simulink model "Final_System_Model_V10"  (R2018a)
settings: Solver=VariableStepAuto  StartTime=0  StopTime=250  FixedStep=0.5  RelTol=1e-3
PreLoadFcn:
  | Ts_Power=1e-6;
  | Ts_Control=100e-6;
undefined symbols (not defined in the file): DiscIntNeverNeededParam, sigbuilder_block
libraries: simulink x24, fl_lib x16, powerlib x15, nesl_utility x8, powerlib_meascontrol x5, re_lib x1
(part 8 of 8)

== system Final_System_Model_V10/Full System/Electrolysers/260 KW Electrolyzer Stack_1/electrolyser stack/electrolyser cell/Eta_B/segma_B/Beta ==
  In1 : Inport
  In2 : Inport  Port=2
  Add3 : Sum
  Add4 : Sum  Inputs=-+
  Add5 : Sum  Inputs=+-
  Add6 : Sum  Inputs=-+
  Constant3 : Constant
  Constant4 : Constant  Value=4
  Constant5 : Constant  Value=2
  Math Function1 : Math  Operator=square  SaturateOnIntegerOverflow=on
  Product5 : Product  Inputs=***
  Product6 : Product  Inputs=*/
  Product7 : Product  Inputs=*/
  Product8 : Product  Inputs=**
  Sqrt : Sqrt  SaturateOnIntegerOverflow=on
  Out1 : Outport
  wires:
  Math Function1/1 -> Add4/2
  Constant3/1 -> Product6/1, Add5/1, Add3/1
  Add3/1 -> Add6/2, Math Function1/1
  Sqrt/1 -> Add6/1
  Constant4/1 -> Product5/1
  Constant5/1 -> Product8/2
  Add4/1 -> Sqrt/1
  Product6/1 -> Add5/2
  Product5/1 -> Add4/1
  Add6/1 -> Product7/1
  Product8/1 -> Product7/2
  Product7/1 -> Out1/1
  In1/1 -> Product5/2, Add3/2
  In2/1 -> Product6/2
  Add5/1 -> Product8/1, Product5/3

== system Final_System_Model_V10/Full System/Electrolysers/260 KW Electrolyzer Stack_1/electrolyser stack/electrolyser cell/Eta_B/segma_B/K_a ==
  In1 : Inport
  In2 : Inport  Port=2
  In3 : Inport  Port=3
  Add2 : Sum  Inputs=+-
  Constant : Constant  Value=-523000
  Constant1 : Constant
  Math Function : Math  SaturateOnIntegerOverflow=on
  Product2 : Product  Inputs=*/
  Product3 : Product  Inputs=*/
  Product4 : Product
  Out1 : Outport
  Out2 : Outport  Port=2
  wires:
  Product4/1 -> Math Function/1
  Add2/1 -> Out2/1, Product4/2
  Math Function/1 -> Out1/1
  In3/1 -> Add2/2
  In2/1 -> Product3/2
  Product2/1 -> Product4/1
  Constant1/1 -> Product3/1
  Product3/1 -> Add2/1
  Constant/1 -> Product2/1
  In1/1 -> Product2/2

== system Final_System_Model_V10/Full System/Electrolysers/260 KW Electrolyzer Stack_1/electrolyser stack/electrolyser cell/Eta_B/segma_B/eta_B ==
  In1 : Inport
  In2 : Inport  Port=2
  Add : Sum
  Product : Product  Inputs=*/
  Out1 : Outport
  wires:
  Product/1 -> Out1/1
  In2/1 -> Add/2
  In1/1 -> Product/1, Add/1
  Add/1 -> Product/2

== system Final_System_Model_V10/Full System/Electrolysers/260 KW Electrolyzer Stack_1/electrolyser stack/electrolyser cell/Eta_B/segma_B/eta_B0 ==
  In1 : Inport
  In2 : Inport  Port=2
  Add1 : Sum
  Product1 : Product  Inputs=/*
  Out1 : Outport
  wires:
  Add1/1 -> Product1/1
  Product1/1 -> Out1/1
  In1/1 -> Add1/1
  In2/1 -> Product1/2, Add1/2

== system Final_System_Model_V10/Full System/Electrolysers/260 KW Electrolyzer Stack_1/electrolyser stack/electrolyser cell/eta_a/n_a/i_a0 ==
  In1 : Inport
  In2 : Inport  Port=2
  Divide : Product  Inputs=*/
  E_a : Constant  Value=76
  Exp : Math  SaturateOnIntegerOverflow=on
  Gain : Gain  Gain=-1
  Multiply : Product
  Multiply1 : Product  Inputs=3
  i_a0ref : Constant  Value=5e-12
  lamda_ma : Subsystem
  Out1 : Outport
  wires:
  Gain/1 -> Exp/1
  Exp/1 -> Multiply1/3
  Multiply/1 -> Gain/1
  Divide/1 -> Multiply/1
  i_a0ref/1 -> Multiply1/1
  In2/1 -> Multiply/2
  Multiply1/1 -> Out1/1
  E_a/1 -> Divide/1
  lamda_ma/1(Out1) -> Multiply1/2
  In1/1 -> Divide/2

== system Final_System_Model_V10/Full System/Electrolysers/260 KW Electrolyzer Stack_1/electrolyser stack/electrolyser cell/eta_c/n_c/i_c0 ==
  In1 : Inport
  In2 : Inport  Port=2
  Divide : Product  Inputs=*/
  E_c : Constant  Value=4.3
  Exp : Math  SaturateOnIntegerOverflow=on
  Gain : Gain  Gain=-1
  Multiply : Product  Inputs=3
  Multiply1 : Product
  i_c0ref : Constant  Value=1e-3
  lamda_mc : Subsystem
  Out1 : Outport
  wires:
  i_c0ref/1 -> Multiply/2
  Multiply/1 -> Out1/1
  Divide/1 -> Multiply1/2
  Multiply1/1 -> Gain/1
  E_c/1 -> Divide/1
  In1/1 -> Divide/2
  lamda_mc/1(Out1) -> Multiply/1
  Exp/1 -> Multiply/3
  Gain/1 -> Exp/1
  In2/1 -> Multiply1/1

== system Final_System_Model_V10/Full System/Electrolysers/93 KW Electrolyzer Stack_2/electrolyser stack/electrolyser cell/Eta_B/segma_B/Beta ==
  In1 : Inport
  In2 : Inport  Port=2
  Add3 : Sum
  Add4 : Sum  Inputs=-+
  Add5 : Sum  Inputs=+-
  Add6 : Sum  Inputs=-+
  Constant3 : Constant
  Constant4 : Constant  Value=4
  Constant5 : Constant  Value=2
  Math Function1 : Math  Operator=square  SaturateOnIntegerOverflow=on
  Product5 : Product  Inputs=***
  Product6 : Product  Inputs=*/
  Product7 : Product  Inputs=*/
  Product8 : Product  Inputs=**
  Sqrt : Sqrt  SaturateOnIntegerOverflow=on
  Out1 : Outport
  wires:
  Add5/1 -> Product5/3, Product8/1
  In2/1 -> Product6/2
  In1/1 -> Add3/2, Product5/2
  Product7/1 -> Out1/1
  Product8/1 -> Product7/2
  Add6/1 -> Product7/1
  Product5/1 -> Add4/1
  Product6/1 -> Add5/2
  Add4/1 -> Sqrt/1
  Constant5/1 -> Product8/2
  Constant4/1 -> Product5/1
  Sqrt/1 -> Add6/1
  Add3/1 -> Math Function1/1, Add6/2
  Constant3/1 -> Add3/1, Add5/1, Product6/1
  Math Function1/1 -> Add4/2

== system Final_System_Model_V10/Full System/Electrolysers/93 KW Electrolyzer Stack_2/electrolyser stack/electrolyser cell/Eta_B/segma_B/K_a ==
  In1 : Inport
  In2 : Inport  Port=2
  In3 : Inport  Port=3
  Add2 : Sum  Inputs=+-
  Constant : Constant  Value=-523000
  Constant1 : Constant
  Math Function : Math  SaturateOnIntegerOverflow=on
  Product2 : Product  Inputs=*/
  Product3 : Product  Inputs=*/
  Product4 : Product
  Out1 : Outport
  Out2 : Outport  Port=2
  wires:
  In1/1 -> Product2/2
  Constant/1 -> Product2/1
  Product3/1 -> Add2/1
  Constant1/1 -> Product3/1
  Product2/1 -> Product4/1
  In2/1 -> Product3/2
  In3/1 -> Add2/2
  Math Function/1 -> Out1/1
  Add2/1 -> Product4/2, Out2/1
  Product4/1 -> Math Function/1

== system Final_System_Model_V10/Full System/Electrolysers/93 KW Electrolyzer Stack_2/electrolyser stack/electrolyser cell/Eta_B/segma_B/eta_B ==
  In1 : Inport
  In2 : Inport  Port=2
  Add : Sum
  Product : Product  Inputs=*/
  Out1 : Outport
  wires:
  Add/1 -> Product/2
  In1/1 -> Add/1, Product/1
  In2/1 -> Add/2
  Product/1 -> Out1/1

== system Final_System_Model_V10/Full System/Electrolysers/93 KW Electrolyzer Stack_2/electrolyser stack/electrolyser cell/Eta_B/segma_B/eta_B0 ==
  In1 : Inport
  In2 : Inport  Port=2
  Add1 : Sum
  Product1 : Product  Inputs=/*
  Out1 : Outport
  wires:
  In2/1 -> Add1/2, Product1/2
  In1/1 -> Add1/1
  Product1/1 -> Out1/1
  Add1/1 -> Product1/1

== system Final_System_Model_V10/Full System/Electrolysers/93 KW Electrolyzer Stack_2/electrolyser stack/electrolyser cell/eta_a/n_a/i_a0 ==
  In1 : Inport
  In2 : Inport  Port=2
  Divide : Product  Inputs=*/
  E_a : Constant  Value=76
  Exp : Math  SaturateOnIntegerOverflow=on
  Gain : Gain  Gain=-1
  Multiply : Product
  Multiply1 : Product  Inputs=3
  i_a0ref : Constant  Value=5e-12
  lamda_ma : Subsystem
  Out1 : Outport
  wires:
  In1/1 -> Divide/2
  lamda_ma/1(Out1) -> Multiply1/2
  E_a/1 -> Divide/1
  Multiply1/1 -> Out1/1
  In2/1 -> Multiply/2
  i_a0ref/1 -> Multiply1/1
  Divide/1 -> Multiply/1
  Multiply/1 -> Gain/1
  Exp/1 -> Multiply1/3
  Gain/1 -> Exp/1

== system Final_System_Model_V10/Full System/Electrolysers/93 KW Electrolyzer Stack_2/electrolyser stack/electrolyser cell/eta_c/n_c/i_c0 ==
  In1 : Inport
  In2 : Inport  Port=2
  Divide : Product  Inputs=*/
  E_c : Constant  Value=4.3
  Exp : Math  SaturateOnIntegerOverflow=on
  Gain : Gain  Gain=-1
  Multiply : Product  Inputs=3
  Multiply1 : Product
  i_c0ref : Constant  Value=1e-3
  lamda_mc : Subsystem
  Out1 : Outport
  wires:
  In2/1 -> Multiply1/1
  Gain/1 -> Exp/1
  Exp/1 -> Multiply/3
  lamda_mc/1(Out1) -> Multiply/1
  In1/1 -> Divide/2
  E_c/1 -> Divide/1
  Multiply1/1 -> Gain/1
  Divide/1 -> Multiply1/2
  Multiply/1 -> Out1/1
  i_c0ref/1 -> Multiply/2

== system Final_System_Model_V10/Full System/Subsystem1/100KW Fuel Cell Stack_2/Fuel Cell Model/ From Current Density (A//cm^2) To Overvoltages (V)/Concentration Overvoltage/IF Function/If Action Subsystem ==
  In1 : Inport
  Action Port : ActionPort  ActionType=then
  Math Function1 : Math  Operator=log  OutputSignalType=real  SaturateOnIntegerOverflow=on
  Out1 : Outport
  wires:
  In1/1 -> Math Function1/1
  Math Function1/1 -> Out1/1

== system Final_System_Model_V10/Full System/Subsystem1/100KW Fuel Cell Stack_2/Fuel Cell Model/ From Current Density (A//cm^2) To Overvoltages (V)/Concentration Overvoltage/IF Function/If Action Subsystem1 ==
  Action Port : ActionPort  ActionType=else
  Constant1 : Constant  Value=0
  Out1 : Outport
  wires:
  Constant1/1 -> Out1/1

== system Final_System_Model_V10/Full System/Subsystem1/100KW Fuel Cell Stack_2/Fuel Cell Model/From Pressures (atm) To Nernest Voltage (V)/From Partial Pressures (atm) To Nernest Voltage (V)/IF Function/If Action Subsystem ==
  In1 : Inport
  Action Port : ActionPort  ActionType=then
  Out1 : Outport
  wires:
  In1/1 -> Out1/1

== system Final_System_Model_V10/Full System/Subsystem1/100KW Fuel Cell Stack_2/Fuel Cell Model/From Pressures (atm) To Nernest Voltage (V)/From Partial Pressures (atm) To Nernest Voltage (V)/IF Function/If Action Subsystem1 ==
  In1 : Inport
  Action Port : ActionPort  ActionType=else
  Out1 : Outport
  wires:
  In1/1 -> Out1/1

== system Final_System_Model_V10/Full System/Subsystem1/80KW Fuel Cell Stack_1/Fuel Cell Model/ From Current Density (A//cm^2) To Overvoltages (V)/Concentration Overvoltage/IF Function/If Action Subsystem ==
  In1 : Inport
  Action Port : ActionPort  ActionType=then
  Math Function1 : Math  Operator=log  OutputSignalType=real  SaturateOnIntegerOverflow=on
  Out1 : Outport
  wires:
  Math Function1/1 -> Out1/1
  In1/1 -> Math Function1/1

== system Final_System_Model_V10/Full System/Subsystem1/80KW Fuel Cell Stack_1/Fuel Cell Model/ From Current Density (A//cm^2) To Overvoltages (V)/Concentration Overvoltage/IF Function/If Action Subsystem1 ==
  Action Port : ActionPort  ActionType=else
  Constant1 : Constant  Value=0
  Out1 : Outport
  wires:
  Constant1/1 -> Out1/1

== system Final_System_Model_V10/Full System/Subsystem1/80KW Fuel Cell Stack_1/Fuel Cell Model/From Pressures (atm) To Nernest Voltage (V)/From Partial Pressures (atm) To Nernest Voltage (V)/IF Function/If Action Subsystem ==
  In1 : Inport
  Action Port : ActionPort  ActionType=then
  Out1 : Outport
  wires:
  In1/1 -> Out1/1

== system Final_System_Model_V10/Full System/Subsystem1/80KW Fuel Cell Stack_1/Fuel Cell Model/From Pressures (atm) To Nernest Voltage (V)/From Partial Pressures (atm) To Nernest Voltage (V)/IF Function/If Action Subsystem1 ==
  In1 : Inport
  Action Port : ActionPort  ActionType=else
  Out1 : Outport
  wires:
  In1/1 -> Out1/1

== system Final_System_Model_V10/Full System/Electrolysers/260 KW Electrolyzer Stack_1/electrolyser stack/electrolyser cell/eta_a/n_a/i_a0/lamda_ma ==
  Constant : Constant  Value=6
  Divide : Product  Inputs=*/
  Gain : Gain  Gain=0.75
  Product : Product
  Product1 : Product
  d_ma : Constant  Value=2.9
  m_Ma : Constant  Value=1e-3
  rho_ma : Constant  Value=22.56
  Out1 : Outport
  wires:
  Gain/1 -> Product1/1
  Divide/1 -> Product1/2
  m_Ma/1 -> Gain/1
  d_ma/1 -> Product/2
  rho_ma/1 -> Product/1
  Product/1 -> Divide/2
  Constant/1 -> Divide/1
  Product1/1 -> Out1/1

== system Final_System_Model_V10/Full System/Electrolysers/260 KW Electrolyzer Stack_1/electrolyser stack/electrolyser cell/eta_c/n_c/i_c0/lamda_mc ==
  Constant : Constant  Value=6
  Divide : Product  Inputs=*/
  Gain : Gain  Gain=0.75
  Multiply : Product
  Multiply1 : Product
  d_mc : Constant  Value=2.7
  m_Mc : Constant  Value=0.3e-3
  rho_mc : Constant  Value=21.45
  Out1 : Outport
  wires:
  Gain/1 -> Multiply1/1
  Divide/1 -> Multiply1/2
  m_Mc/1 -> Gain/1
  Constant/1 -> Divide/1
  d_mc/1 -> Multiply/2
  Multiply/1 -> Divide/2
  Multiply1/1 -> Out1/1
  rho_mc/1 -> Multiply/1

== system Final_System_Model_V10/Full System/Electrolysers/93 KW Electrolyzer Stack_2/electrolyser stack/electrolyser cell/eta_a/n_a/i_a0/lamda_ma ==
  Constant : Constant  Value=6
  Divide : Product  Inputs=*/
  Gain : Gain  Gain=0.75
  Product : Product
  Product1 : Product
  d_ma : Constant  Value=2.9
  m_Ma : Constant  Value=1e-3
  rho_ma : Constant  Value=22.56
  Out1 : Outport
  wires:
  Product1/1 -> Out1/1
  Constant/1 -> Divide/1
  Product/1 -> Divide/2
  rho_ma/1 -> Product/1
  d_ma/1 -> Product/2
  m_Ma/1 -> Gain/1
  Divide/1 -> Product1/2
  Gain/1 -> Product1/1

== system Final_System_Model_V10/Full System/Electrolysers/93 KW Electrolyzer Stack_2/electrolyser stack/electrolyser cell/eta_c/n_c/i_c0/lamda_mc ==
  Constant : Constant  Value=6
  Divide : Product  Inputs=*/
  Gain : Gain  Gain=0.75
  Multiply : Product
  Multiply1 : Product
  d_mc : Constant  Value=2.7
  m_Mc : Constant  Value=0.3e-3
  rho_mc : Constant  Value=21.45
  Out1 : Outport
  wires:
  rho_mc/1 -> Multiply/1
  Multiply1/1 -> Out1/1
  Multiply/1 -> Divide/2
  d_mc/1 -> Multiply/2
  Constant/1 -> Divide/1
  m_Mc/1 -> Gain/1
  Divide/1 -> Multiply1/2
  Gain/1 -> Multiply1/1

== stateflow chart Final_System_Model_V10/Full System/Chart1 ==
  state LOAD [parallel]
    settings: executionOrder=1
    state LOAD_OFF
      entry: load_on=0;
    state LOAD_ON
      entry: load_on=1;
    (default) -> LOAD_OFF
    LOAD_OFF -> LOAD_ON : [load>0]
    LOAD_ON -> LOAD_OFF : [~load>0]
  state Battery [parallel]
    settings: executionOrder=5
    state Battery_Isolated
      entry: pvtobattery=0;
      entry: batterytoload =0;
    state Battery_Charging
      entry: pvtobattery=1;
    state Battery_Discharging
      entry:batterytoload =1;
      exit:batterytoload=0;
    (default) -> Battery_Isolated
    Battery_Charging -> Battery_Isolated [order 1] : [(battery_full==1) && (delta<0) ]
    Battery_Isolated -> Battery_Charging [order 2] : [(battery_full==0) && (delta<0) ]
    Battery_Discharging -> Battery_Charging [order 1] : [[delta<0 && battery_full==0]]
    Battery_Charging -> Battery_Discharging [order 2] : [[(delta>0 && delta<=72) || (delta>=88 && delta<=90) || (delta>=110 && delta<=162) || (delta>=198 && delta<=215) ]]
    Battery_Discharging -> Battery_Isolated [order 2] : [delta<0 || battery_empty==1 || (delta>72 && delta<88) || (delta>90 && delta<110) || (delta>162 && delta<198)]
    Battery_Isolated -> Battery_Discharging [order 1] : [(delta>0 && delta<=72) || (delta>=88 && delta<=90) || (delta>=110 && delta<=162) || (delta>=198 && delta<=215) ]
  state Electrolyser_1 [parallel]
    settings: executionOrder=4
    state Electrolyser_1_OFF
      entry: pvtoelec_1=0;
    state Electrolyser_1_ON
      entry: pvtoelec_1=1;
    (default) -> Electrolyser_1_OFF
    Electrolyser_1_OFF -> Electrolyser_1_ON : [delta<0 && battery_full==1 && tank_full==0]
    Electrolyser_1_ON -> Electrolyser_1_OFF : [delta>=0 || tank_full==1]
  state Electrolyser_2 [parallel]
    settings: executionOrder=6
    state Electrolyser_2_OFF
      entry: pvtoelec_2=0;
    state Electrolyser_2_ON
      entry: pvtoelec_2=1;
    (default) -> Electrolyser_2_OFF
    Electrolyser_2_OFF -> Electrolyser_2_ON : [delta<-260 && battery_full==1 && tank_full==0]
    Electrolyser_2_ON -> Electrolyser_2_OFF : [delta>=0 || tank_full==1]
  state FC_1 [parallel]
    settings: executionOrder=2
    state FC_1_OFF
      entry: fctoload_1=0;
    state FC_1_ON
      entry: fctoload_1=1;
    (default) -> FC_1_OFF
    FC_1_OFF -> FC_1_ON : [(delta>72 && delta<88) || (delta>=88 && delta<90) || (delta>162 && delta<198) || (delta>=198 && delta<215) || delta>215 ]
    FC_1_ON -> FC_1_OFF : [delta<=1 || (delta<=72 && delta>1) || (delta>=90 && delta<=162)]
  state FC_2 [parallel]
    settings: executionOrder=3
    state FC_2_OFF
      entry: fctoload_2=0;
    state FC_2_ON
      entry: fctoload_2=1;
    (default) -> FC_2_OFF
    FC_2_OFF -> FC_2_ON : [(delta>90 && delta<110) || (delta>=110 && delta<162) || (delta>198 && delta<215) || delta>215]
    FC_2_ON -> FC_2_OFF : [delta<=1 || (delta<=90 && delta>1) || ( delta>=162 && delta<=198)]
  state tank [parallel]
    settings: executionOrder=7
    state tank_Charging
      entry:elect_1totank=1;
      elect_2totank=1;
    state tank_Isolated
      entry: tanktofc_1=0;
      tanktofc_2 =0;
      elect_1totank=0;
      elect_2totank=0;
    state tank_Discharging
      entry:tanktofc_1=1;
      tanktofc_2=1;
    (default) -> tank_Isolated
    tank_Isolated -> tank_Charging [order 2] : [(pvtoelec_1==1 || pvtoelec_2==1)]
    tank_Charging -> tank_Isolated [order 2] : [(pvtoelec_1==0 && pvtoelec_2==0)]
    tank_Discharging -> tank_Charging [order 1] : [pvtoelec_1==1||pvtoelec_2==1]
    tank_Charging -> tank_Discharging [order 1] : [pvtoelec_1==0&&pvtoelec_2==0]
    tank_Discharging -> tank_Isolated [order 2] : [fctoload_1==0&&fctoload_2==0]
    tank_Isolated -> tank_Discharging [order 1] : [fctoload_1==1||fctoload_2==1]
  data: battery_full function_input; tank_full function_input; delta2 function_input; fc1toload_on function_output; fc2toload_on function_output; pvtoload_on function_output; batterytoload_on function_output; pvtobattery_on function_output; pvtoelectrolyser_on function_output; load_on output; battery_full1 input; tank_full1 input; delta input; load input; fctoload_1 output; battery_full input; tank_full input; fctoload_2 output; pvtoelec_1 output; pvtobattery output; batterytoload output; battery_empty input; pvtoelec_2 output; tanktofc_1 output; tanktofc_2 output; elect_1totank output; elect_2totank output
  function [fc1toload_on,fc2toload_on,pvtoload_on,batterytoload_on,pvtobattery_on,pvtoelectrolyser_on] = Operation(battery_full, tank_full, delta2):
    | function [fc1toload_on,fc2toload_on,pvtoload_on,batterytoload_on,pvtobattery_on,pvtoelectrolyser_on] = Operation(battery_full, tank_full, delta2)
    | 
    | aVarTruthTableCondition_1 = false;
    | aVarTruthTableCondition_2 = false;
    | aVarTruthTableCondition_3 = false;
    | aVarTruthTableCondition_4 = false;
    | aVarTruthTableCondition_5 = false;
    | aVarTruthTableCondition_6 = false;
    | aVarTruthTableCondition_7 = false;
    | aVarTruthTableCondition_8 = false;
    | aVarTruthTableCondition_9 = false;
    | aVarTruthTableCondition_10 = false;
    | aVarTruthTableCondition_11 = false;
    | 
    | 
    | % Excess Power
    | 
    | aVarTruthTableCondition_1 = logical(delta<0);
    | 
    | % Battery Full
    | 
    | aVarTruthTableCondition_2 = logical(battery_full==1);
    | 
    | % Tank Full
    | 
    | aVarTruthTableCondition_3 = logical(tank_full==1);
    | 
    | % PV meets Demand
    | 
    | aVarTruthTableCondition_4 = logical(delta==0);
    | 
    | % Shortage1
    | % Battery ON Only
    | 
    | aVarTruthTableCondition_5 = logical(delta<72);
    | 
    | % Shortage2
    | % FC1 Only
    | 
    | aVarTruthTableCondition_6 = logical(delta<88);
    | 
    | % Shortage3
    | % FC1 + Battery
    | 
    | aVarTruthTableCondition_7 = logical(delta<90);
    | 
    | % Shortage4
    | % FC2 Only
    | 
    | aVarTruthTableCondition_8 = logical(delta<110);
    | 
    | % Shortage5
    | %  FC2 + Battery
    | 
    | aVarTruthTableCondition_9 = logical(delta<162);
    | 
    | % Shortage6
    | % FC1 + FC2
    | 
    | aVarTruthTableCondition_10 = logical(delta<198);
    | 
    | % Shortage7
    | % FC1 +FC2 + Battery
    | 
    | aVarTruthTableCondition_11 = logical(delta<214);
    | 
    | if (aVarTruthTableCondition_1 && ~aVarTruthTableCondition_2)
    |     A1();
    | elseif (aVarTruthTableCondition_1 && aVarTruthTableCondition_2 && ~aVarTruthTableCondition_3)
    |     A2();
    | elseif (aVarTruthTableCondition_4)
    |     A3();
    | elseif (~aVarTruthTableCondition_4 && aVarTruthTableCondition_5)
    |     A4();
    | elseif (~aVarTruthTableCondition_5 && aVarTruthTableCondition_6)
    |     A5();
    | elseif (~aVarTruthTableCondition_6 && aVarTruthTableCondition_7)
    |     A6();
    | elseif (~aVarTruthTableCondition_7 && aVarTruthTableCondition_8)
    |     A7();
    | elseif (~aVarTruthTableCondition_8 && aVarTruthTableCondition_9)
    |     A8();
    | elseif (~aVarTruthTableCondition_9 && aVarTruthTableCondition_10)
    |     A9();
    | elseif (~aVarTruthTableCondition_10 && aVarTruthTableCondition_11)
    |     A10();
    | elseif (aVarTruthTableCondition_1 && aVarTruthTableCondition_2 && aVarTruthTableCondition_3)
    |     A11();
    | else % Default
    |     DA();
    | end
    | 
    | function A1()
    | 
    | % Excess Power ِAND Battery Empty
    | 
    | fc1toload_on=0;
    | fc2toload_on=0;
    | pvtoload_on=1;
    | batterytoload_on=0;
    | pvtobattery_on=1;
    | pvtoelectrolyser_on=0;
    | 
    | function A2()
    | 
    | % Excess power AND Battery Full AND Tank Empty
    | 
    | fc1toload_on=0;
    | fc2toload_on=0;
    | pvtoload_on=1;
    | batterytoload_on=0;
    | pvtobattery_on=0;
    | pvtoelectrolyser_on=1;
    | 
    | function A3()
    | 
    | % PV meets Demand
    | 
    | fc1toload_on=0;
    | fc2toload_on=0;
    | pvtoload_on=1;
    | batterytoload_on=0;
    | pvtobattery_on=0;
    | pvtoelectrolyser_on=0;
    | 
    | function A4()
    | 
    | % Shortage1
    | % Battery ON Only
    | 
    | fc1toload_on=0;
    | fc2toload_on=0;
    | pvtoload_on=1;
    | batterytoload_on=1;
    | pvtobattery_on=0;
    | pvtoelectrolyser_on=0;
    | 
    | function A5()
    | 
    | % Shortage2
    | % FC1 Only
    | 
    | fc1toload_on=1;
    | fc2toload_on=0;
    | pvtoload_on=1;
    | batterytoload_on=0;
    | pvtobattery_on=0;
    | pvtoelectrolyser_on=0;
    | 
    | function A6()
    | 
    | % Shortage3
    | % FC1 + Battery
    | 
    | fc1toload_on=1;
    | fc2toload_on=0;
    | pvtoload_on=1;
    | batterytoload_on=1;
    | pvtobattery_on=0;
    | pvtoelectrolyser_on=0;
    | 
    | function A7()
    | 
    | % Shortage4
    | % FC2 Only
    | 
    | fc1toload_on=0;
    | fc2toload_on=1;
    | pvtoload_on=1;
    | batterytoload_on=0;
    | pvtobattery_on=0;
    | pvtoelectrolyser_on=0;
    | 
    | function A8()
    | 
    | % Shortage5
    | %  FC2 + Battery
    | 
    | fc1toload_on=0;
    | fc2toload_on=1;
    | pvtoload_on=1;
    | batterytoload_on=1;
    | pvtobattery_on=0;
    | pvtoelectrolyser_on=0;
    | 
    | function A9()
    | 
    | % Shortage6
    | % FC1 + FC2
    | 
    | fc1toload_on=1;
    | fc2toload_on=1;
    | pvtoload_on=1;
    | batterytoload_on=0;
    | pvtobattery_on=0;
    | pvtoelectrolyser_on=0;
    | 
    | function A10()
    | 
    | % Shortage7
    | % FC1 +FC2 + Battery
    | 
    | fc1toload_on=1;
    | fc2toload_on=1;
    | pvtoload_on=1;
    | batterytoload_on=1;
    | pvtobattery_on=0;
    | pvtoelectrolyser_on=0;
    | 
    | function DA()
    | 
    | % Default
    | 
    | fc1toload_on=0;
    | fc2toload_on=0;
    | pvtoload_on=0;
    | batterytoload_on=0;
    | pvtobattery_on=0;
    | pvtoelectrolyser_on=0;
    | 
    | function A11()
    | 
    | % Excess Power AND Battery Full AND Tank Full
    | 
    | fc1toload_on=0;
    | fc2toload_on=0;
    | pvtoload_on=1;
    | batterytoload_on=0;
    | pvtobattery_on=0;
    | pvtoelectrolyser_on=0;
